simulink model "hdlFrame_HarrisCornerDetection_2D_NPSS"  (R2023a)
settings: Solver=FixedStepDiscrete  StartTime=0.0  StopTime=0  RelTol=1e-3
InitFcn:
  | slfeature('SLBlockSimThruCGXE', 2);
  | slfeature('SLCGEVCGDomainSubsystem', 1);
model workspace (MAT data in the model file):
  h = 5
  im = [0.16862745098 0.172549019608 0.16862745098 0.16862745098 0.172549019608 0.176470588235 0.16862745098 0.172549019608 0.172549019608 0.164705882353 0.160784313725 0.164705882353 ... (196608 elements, 384x512)]
  w = 5
undefined symbols (not defined in the file or in its folder): checkerboard, gray
(part 1 of 2)
settings Model: SimulationMode=software-in-the-loop (sil)  Creator=mcao  LastModifiedBy=navan
settings SolverCC: AlgebraicLoopSolver=TrustRegion  MaxZcPerStep=1
settings DataIOCC: SaveFormat=StructureWithTime  SignalLogging=off  DSMLogging=off
settings OptimizationCC: DefaultParameterBehavior=Inlined  ReuseModelBlockBuffer=off  EnhancedBackFolding=on  PassReuseOutputArgsAs=Individual arguments  RollThreshold=15  ZeroExternalMemoryAtStartup=off  ZeroInternalMemoryAtStartup=off  OptimizeBlockOrder=speed  DifferentSizesBufferReuse=on  OptimizationCustomize=off  EfficientTunableParamExpr=on
settings DebuggingCC: ParameterTunabilityLossMsg=error  UnconnectedInputMsg=warning  UnconnectedOutputMsg=warning  UnconnectedLineMsg=warning  ModelReferenceSymbolNameMessage=none
settings HardwareCC: ProdBitPerPointer=32  ProdBitPerSizeT=32  ProdBitPerPtrDiffT=32  ProdLargestAtomicFloat=None  ProdWordSize=32  ProdHWDeviceType=Custom Processor->Custom Processor  TargetBitPerLong=64  TargetBitPerPointer=64  TargetBitPerSizeT=64  TargetBitPerPtrDiffT=64  TargetLongLongMode=on  TargetIntDivRoundTo=Zero  TargetEndianess=LittleEndian  TargetWordSize=64  TargetHWDeviceType=Custom Processor->MATLAB Host Computer  ProdEqTarget=off
settings ModelReferenceCC: EnableRefExpFcnMdlSchedulingChecks=on
settings SFSimCC: MATLABDynamicMemAlloc=off
settings RTWCC: Description=Embedded Coder  SystemTargetFile=ert.tlc  TemplateMakefile=ert_default_tmf  DLArmComputeVersion=19.05
settings CodeAppCC: ForceParamTrailComments=on  IgnoreCustomStorageClasses=off  OperatorAnnotations=on  SimulinkDataObjDesc=on  SFDataObjDesc=on  InsertBlockDesc=on
settings ERTTargetCC: TargetLangStandard=C99 (ISO)  GenerateSampleERTMain=on  InlinedParameterPlacement=NonHierarchical  ERTCustomFileTemplate=example_file_process.tlc

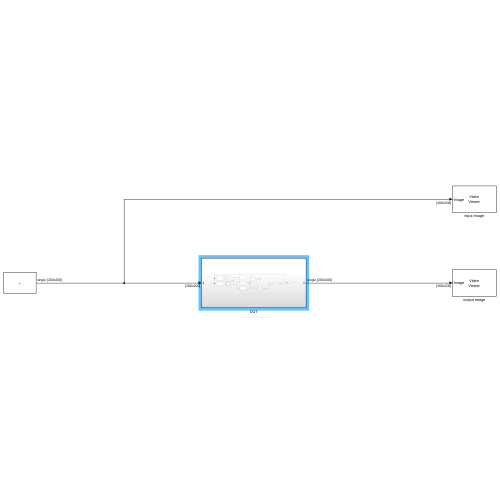
[thumbnail: Simulink's stored preview of the top-level diagram]
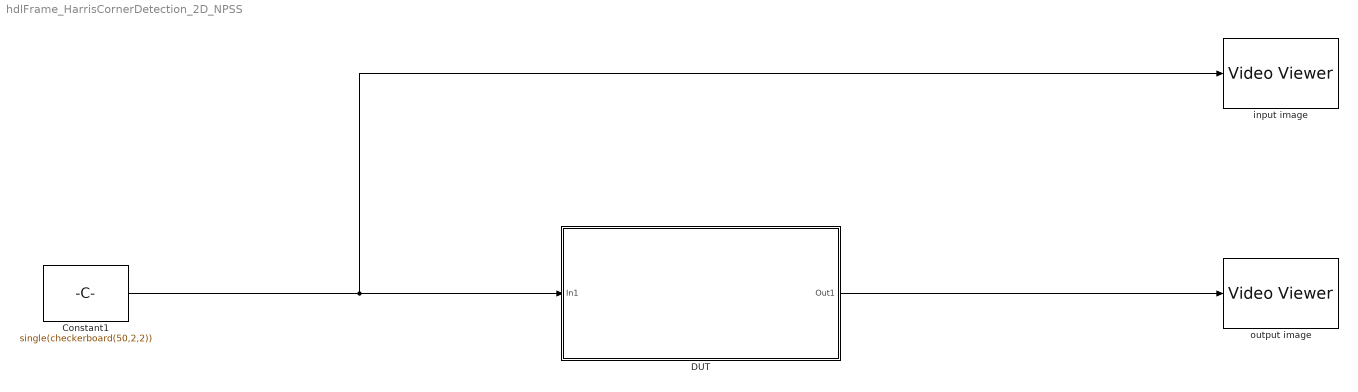
== system hdlFrame_HarrisCornerDetection_2D_NPSS ==
  Constant1 : Constant  Value=single(checkerboard(50,2,2))  SampleTime=1
  DUT : Subsystem
  input image : VideoViewer  colormapValue=gray(256)  FigPos=[408 1010 1280 623]
  output image : VideoViewer  colormapValue=gray(256)  FigPos=[410 803 1281 623]
  wires:
  Constant1/1 -> input image/1, DUT/1(In1)
  DUT/1(Out1) -> output image/1
